simulink library "FOUROSEM_WD_DC_MASTER"  (Simulink 8.0)
settings: Solver=ode45  StartTime=0.0  StopTime=10.0  RelTol=1e-3
libraries: cdsFilt x4, cdsEpicsIn x2
settings Model: Creator=controls  LastModifiedBy=controls

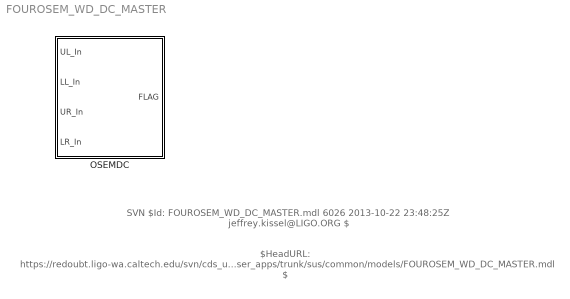
== system FOUROSEM_WD_DC_MASTER ==
  note: $HeadURL: https://redoubt.ligo-wa.caltech.edu/svn/cds_user_apps/trunk/sus/common/models/FOUROSEM_WD_DC_MASTER.mdl $
  note: SVN $Id: FOUROSEM_WD_DC_MASTER.mdl 6026 2013-10-22 23:48:25Z jeffrey.kissel@LIGO.ORG $
  OSEMDC : Subsystem

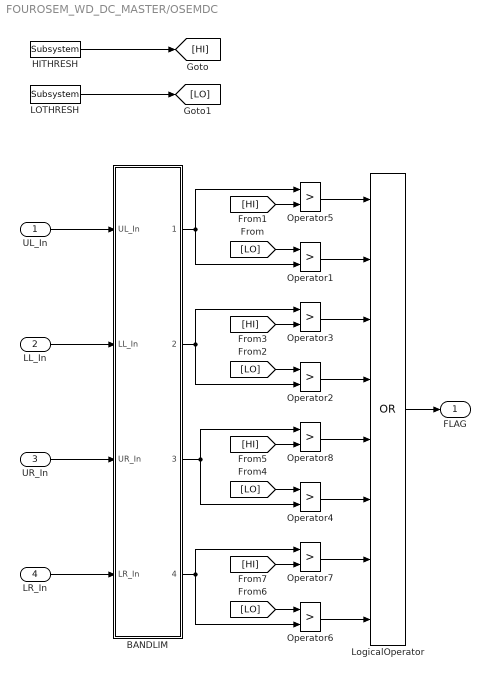
== system FOUROSEM_WD_DC_MASTER/OSEMDC ==
  UL_In : Inport
  LL_In : Inport  Port=2
  UR_In : Inport  Port=3
  LR_In : Inport  Port=4
  BANDLIM : Subsystem
  HITHRESH : cdsEpicsIn/Subsystem  Tag=cdsEpicsIn  Description=|  SystemSampleTime=-1
      | Purpose:                                                                              
      | Create an EPICS input channel connection to the FE realtime controls.                 
      |                                                                                       
      | Operation:                                                                            
      | Outputs value from an EPICS ai record. Value is floating point with a precision of 3..
      |                                                                                       
      | Usage:                                                                                
      | Name the part with the desired EPICS channel name.
      settings: AttributesFormatString=%<Tag>
  LOTHRESH : cdsEpicsIn/Subsystem  Tag=cdsEpicsIn  Description=|  SystemSampleTime=-1
      | Purpose:                                                                              
      | Create an EPICS input channel connection to the FE realtime controls.                 
      |                                                                                       
      | Operation:                                                                            
      | Outputs value from an EPICS ai record. Value is floating point with a precision of 3..
      |                                                                                       
      | Usage:                                                                                
      | Name the part with the desired EPICS channel name.
      settings: AttributesFormatString=%<Tag>
  LogicalOperator : Logic  Operator=OR  Inputs=8  AllPortsSameDT=off  OutDataTypeStr=boolean
  Operator{1..8} (8 alike) : RelationalOperator  Operator=>  OutDataTypeStr=boolean
  FLAG : Outport
  wires:
  UL_In/1 -> BANDLIM/1(UL_In)
  LL_In/1 -> BANDLIM/2(LL_In)
  UR_In/1 -> BANDLIM/3(UR_In)
  LR_In/1 -> BANDLIM/4(LR_In)
  BANDLIM/1(UL_Out) -> Operator5/1, Operator1/2
  Operator5/1 -> LogicalOperator/1
  Operator1/1 -> LogicalOperator/2
  Operator3/1 -> LogicalOperator/3
  Operator2/1 -> LogicalOperator/4
  BANDLIM/2(LL_Out) -> Operator3/1, Operator2/2
  Operator8/1 -> LogicalOperator/5
  Operator4/1 -> LogicalOperator/6
  Operator7/1 -> LogicalOperator/7
  Operator6/1 -> LogicalOperator/8
  BANDLIM/4(LR_Out) -> Operator7/1, Operator6/2
  BANDLIM/3(UR_Out) -> Operator8/1, Operator4/2
  LogicalOperator/1 -> FLAG/1
  HITHRESH/1 -> [HI]
  LOTHRESH/1 -> [LO]
  [HI] -> Operator5/2
  [LO] -> Operator1/1
  [HI] -> Operator3/2
  [LO] -> Operator2/1
  [HI] -> Operator8/2
  [LO] -> Operator4/1
  [HI] -> Operator7/2
  [LO] -> Operator6/1

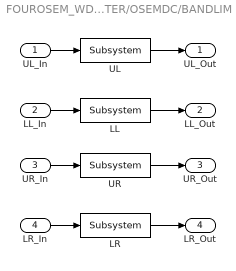
== system FOUROSEM_WD_DC_MASTER/OSEMDC/BANDLIM ==
  UL_In : Inport
  LL_In : Inport  Port=2
  UR_In : Inport  Port=3
  LR_In : Inport  Port=4
  LL : cdsFilt/Subsystem  Tag=cdsFilt  Description=|  SystemSampleTime=-1
      | Purpose:                                                                                                                                                                                                                                  
      | Standard CDS IIR filter module.                                                                                                                                                                                                           
      |                                                                                                                                                                                                                                           
      | Operation:                                                                                                                                                                                                                                
      | Consists of 10 second order section IIR filters, plus a ramped gain stage. In FE code, also provides pre-defined test points and excitation channel inputs. The filter coefficients are defined in the LIGO system using the 'foton' tool.
      |                                                                                                                                                                                                                                           
      | Usage:                                                                                                                                                                                                                                    
      | Name the part with the desired filter module name.
      settings: AttributesFormatString=%<Tag>
  LR : cdsFilt/Subsystem  Tag=cdsFilt  Description=|  SystemSampleTime=-1
      | Purpose:                                                                                                                                                                                                                                  
      | Standard CDS IIR filter module.                                                                                                                                                                                                           
      |                                                                                                                                                                                                                                           
      | Operation:                                                                                                                                                                                                                                
      | Consists of 10 second order section IIR filters, plus a ramped gain stage. In FE code, also provides pre-defined test points and excitation channel inputs. The filter coefficients are defined in the LIGO system using the 'foton' tool.
      |                                                                                                                                                                                                                                           
      | Usage:                                                                                                                                                                                                                                    
      | Name the part with the desired filter module name.
      settings: AttributesFormatString=%<Tag>
  UL : cdsFilt/Subsystem  Tag=cdsFilt  Description=|  SystemSampleTime=-1
      | Purpose:                                                                                                                                                                                                                                  
      | Standard CDS IIR filter module.                                                                                                                                                                                                           
      |                                                                                                                                                                                                                                           
      | Operation:                                                                                                                                                                                                                                
      | Consists of 10 second order section IIR filters, plus a ramped gain stage. In FE code, also provides pre-defined test points and excitation channel inputs. The filter coefficients are defined in the LIGO system using the 'foton' tool.
      |                                                                                                                                                                                                                                           
      | Usage:                                                                                                                                                                                                                                    
      | Name the part with the desired filter module name.
      settings: AttributesFormatString=%<Tag>
  UR : cdsFilt/Subsystem  Tag=cdsFilt  Description=|  SystemSampleTime=-1
      | Purpose:                                                                                                                                                                                                                                  
      | Standard CDS IIR filter module.                                                                                                                                                                                                           
      |                                                                                                                                                                                                                                           
      | Operation:                                                                                                                                                                                                                                
      | Consists of 10 second order section IIR filters, plus a ramped gain stage. In FE code, also provides pre-defined test points and excitation channel inputs. The filter coefficients are defined in the LIGO system using the 'foton' tool.
      |                                                                                                                                                                                                                                           
      | Usage:                                                                                                                                                                                                                                    
      | Name the part with the desired filter module name.
      settings: AttributesFormatString=%<Tag>
  UL_Out : Outport
  LL_Out : Outport  Port=2
  UR_Out : Outport  Port=3
  LR_Out : Outport  Port=4
  wires:
  UL/1 -> UL_Out/1
  LL/1 -> LL_Out/1
  UR/1 -> UR_Out/1
  UL_In/1 -> UL/1
  LL_In/1 -> LL/1
  UR_In/1 -> UR/1
  LR/1 -> LR_Out/1
  LR_In/1 -> LR/1
